simulink model "JT9D_Model_SS_test_with_alti"  (R2016b)
settings: Solver=FixedStepDiscrete  StartTime=0.0  StopTime=30.0  FixedStep=0.2  RelTol=1e-3  EnableMultiTasking=on
values from neighbouring files (symbols this model uses):
  MWS = input_set_0_0_15(MWS)    [JT9D_setup_everything_Dyn.m]    (also in JT9D_setup_everything_SS_test_with_alti.m = setup_Inputs(MWS))
undefined symbols (not defined in the file or in its folder): stripchar_TMATS
libraries: Lib_Turbo_Duct_TMATS x5, Lib_Turbo_Compressor_TMATS x3, Lib_Turbo_Shaft_TMATS x2, Lib_Turbo_TurbineNPSS_TMATS x2, Lib_Turbo_Nozzle_TMATS x2, Lib_Turbo_Ambient_TMATS x1, Lib_Turbo_Burner_TMATS x1, Lib_Turbo_Inlet_TMATS x1, Lib_Turbo_StaticCalc_TMATS x1, Lib_Turbo_SFCCalc_TMATS x1, Lib_Turbo_Splitter_TMATS x1, Lib_Solve_SSNRSolverJC_TMATS x1
settings Model: Creator=jwchapm2  LastModifiedBy=zhangshu
settings DataIOCC: LimitDataPoints=on  SaveFormat=Array
settings OptimizationCC: ExpressionDepthLimit=2147483647  LifeSpan=inf
settings DebuggingCC: UnderspecifiedInitializationDetection=Classic  MergeDetectMultiDrivingBlocksExec=none  SolverPrmCheckMsg=warning  StateNameClashWarn=warning  SFUnexpectedBacktrackingDiag=warning  SFNoUnconditionalDefaultTransitionDiag=warning  SFExecutionAtInitializationDiag=none
settings HardwareCC: ProdBitPerPointer=32  ProdBitPerSizeT=32  ProdBitPerPtrDiffT=32  ProdLargestAtomicFloat=None  ProdIntDivRoundTo=Undefined  ProdEndianess=Unspecified  ProdWordSize=32  ProdHWDeviceType=32-bit Generic
settings ModelReferenceCC: PropagateSignalLabelsOutOfModel=off
settings GRTTargetCC: TargetLangStandard=C89/C90 (ANSI)  GeneratePreprocessorConditionals=Disable all
settings ConfigComp: CovMetricSettings=dw  CovHtmlReporting=on  CovSaveCumulativeToWorkspaceVar=on  CovSaveSingleToWorkspaceVar=on  CovExternalEMLEnable=off

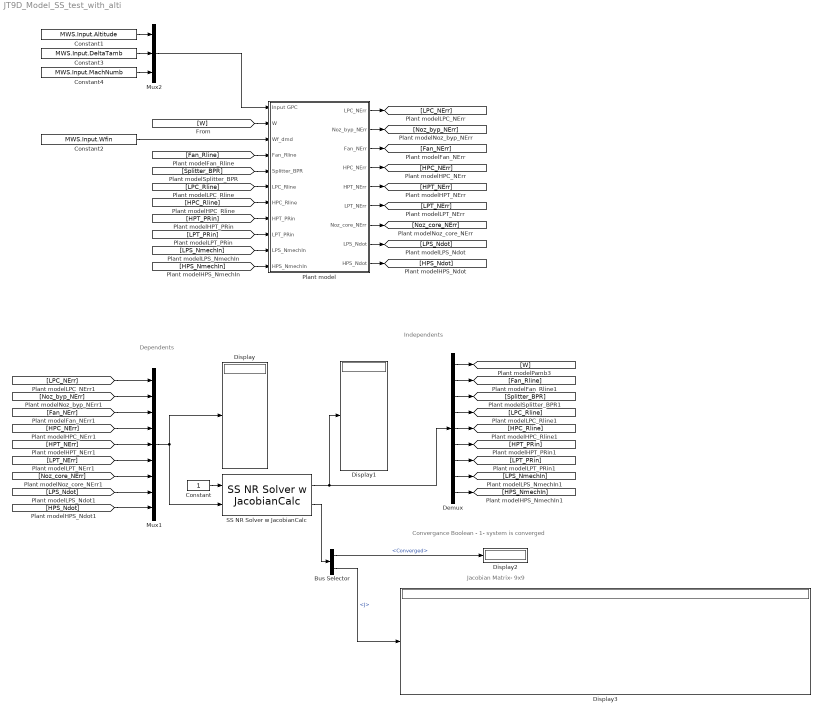
== system JT9D_Model_SS_test_with_alti ==
  note: Jacobian Matrix- 9x9
  note: Dependents
  note: Independents
  note: Convergance Boolean - 1- system is converged
  Bus Selector : BusSelector  OutputSignals=Converged,J
  Constant : Constant
  Constant1 : Constant  Value=MWS.Input.Altitude
  Constant2 : Constant  Value=MWS.Input.Wfin
  Constant3 : Constant  Value=MWS.Input.DeltaTamb
  Constant4 : Constant  Value=MWS.Input.MachNumb
  Demux : Demux  Outputs=9
  Display{,1..3} (4 alike) : Display
  Mux1 : Mux  Inputs=9
  Mux2 : Mux  Inputs=3
  Plant model : Subsystem
  SS NR Solver w JacobianCalc : Lib_Solve_SSNRSolverJC_TMATS/SS NR Solver w JacobianCalc  SJac_Per_M=0.01*[ones(size(MWS.Input.NRIC,2),1)'; -ones(size(MWS.Input.NRIC,2),1)']  SNR_IC_M=MWS.Input.NRIC  SNR_DX_M=1  SNR_Mx_M=100000  SNR_Mn_M=0.00001  SJacobianAttempts_M=20  Cond_Limits_M=0.005
  wires:
  Constant2/1 -> Plant model/3(Wf_dmd)
  [Fan_Rline] -> Plant model/4(Fan_Rline)
  [Splitter_BPR] -> Plant model/5(Splitter_BPR)
  [HPT_PRin] -> Plant model/8(HPT_PRin)
  [LPT_PRin] -> Plant model/9(LPT_PRin)
  [LPS_NmechIn] -> Plant model/10(LPS_NmechIn)
  [HPS_NmechIn] -> Plant model/11(HPS_NmechIn)
  Plant model/1(LPC_NErr) -> [LPC_NErr]
  Plant model/2(Noz_byp_NErr) -> [Noz_byp_NErr]
  Plant model/3(Fan_NErr) -> [Fan_NErr]
  Plant model/4(HPC_NErr) -> [HPC_NErr]
  Plant model/5(HPT_NErr) -> [HPT_NErr]
  Plant model/6(LPT_NErr) -> [LPT_NErr]
  Plant model/7(Noz_core_NErr) -> [Noz_core_NErr]
  Plant model/8(LPS_Ndot) -> [LPS_Ndot]
  Plant model/9(HPS_Ndot) -> [HPS_Ndot]
  Demux/1 -> [W]
  Demux/7 -> [LPT_PRin]
  Demux/5 -> [HPC_Rline]
  Demux/6 -> [HPT_PRin]
  Demux/4 -> [LPC_Rline]
  Demux/8 -> [LPS_NmechIn]
  Demux/9 -> [HPS_NmechIn]
  Demux/2 -> [Fan_Rline]
  Demux/3 -> [Splitter_BPR]
  [Fan_NErr] -> Mux1/3
  [HPC_NErr] -> Mux1/4
  [Noz_byp_NErr] -> Mux1/2
  [HPT_NErr] -> Mux1/5
  [LPC_NErr] -> Mux1/1
  [LPT_NErr] -> Mux1/6
  [Noz_core_NErr] -> Mux1/7
  SS NR Solver w JacobianCalc/2 -> Bus Selector/1
  Mux1/1 -> SS NR Solver w JacobianCalc/2, Display/1
  Bus Selector/1 -> Display2/1  "<Converged>"
  Bus Selector/2 -> Display3/1  "<J>"
  [LPS_Ndot] -> Mux1/8
  [HPS_Ndot] -> Mux1/9
  SS NR Solver w JacobianCalc/1 -> Demux/1, Display1/1
  Constant/1 -> SS NR Solver w JacobianCalc/1
  [HPC_Rline] -> Plant model/7(HPC_Rline)
  [LPC_Rline] -> Plant model/6(LPC_Rline)
  [W] -> Plant model/2(W)
  Constant1/1 -> Mux2/1
  Constant3/1 -> Mux2/2
  Constant4/1 -> Mux2/3
  Mux2/1 -> Plant model/1(Input GPC)

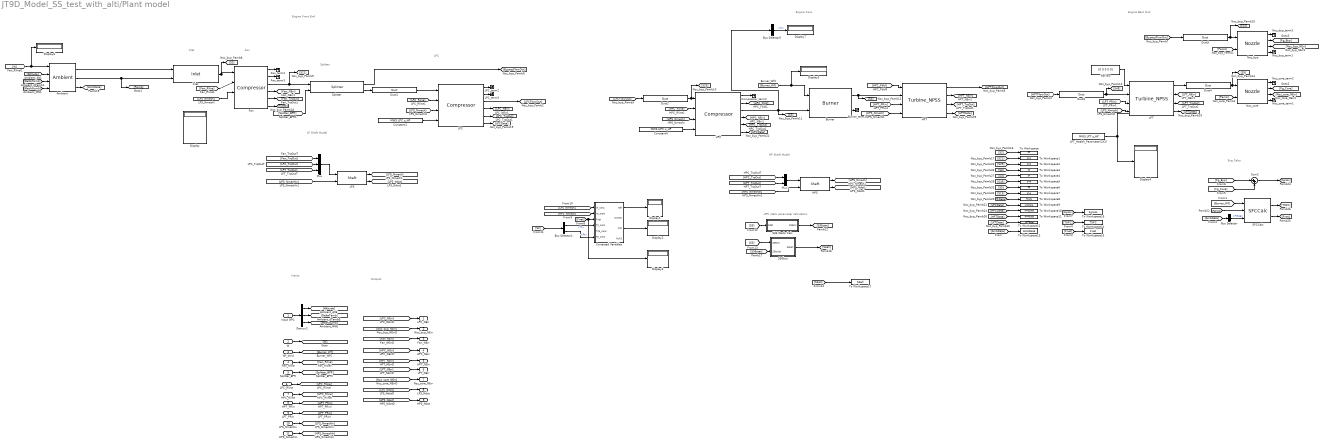
== system JT9D_Model_SS_test_with_alti/Plant model ==
  note: LP Shaft Model
  note: Inputs
  note: Outputs
  note: Engine Core
  note: HP Shaft Model
  note: Engine Back End
  note: Engine Front End
  note: Inlet
  note: Fan
  note: Splitter
  note: LPC
  note: Eng Calcs
  note: HPC static parameter calculation
  Input GPC : Inport
  W : Inport  Port=2
  Wf_dmd : Inport  Port=3
  Fan_Rline : Inport  Port=4
  Splitter_BPR : Inport  Port=5
  LPC_Rline : Inport  Port=6
  HPC_Rline : Inport  Port=7
  HPT_PRin : Inport  Port=8
  LPT_PRin : Inport  Port=9
  LPS_NmechIn : Inport  Port=10
  HPS_NmechIn : Inport  Port=11
  Ambient : Lib_Turbo_Ambient_TMATS/Ambient  X_A_AltVec_M=5000*[-1 0 1 2 3 4 5 6 7 8 9 10 12 14 16]  T_A_TsVec_M=[536.51 518.67 500.84 483.03 465.22 447.41 429.62 411.84 394.06 389.97 389.97 389.97 389.97 392.25 397.69]  T_A_PsVec_M=[17.554 14.696 12.228 10.108 8.297 6.759 5.461 4.373 3.468 2.73 2.149 1.692 1.049 0.651 0.406]  AFARc_M=0  X_A_FARVec_M=[0; 0.0050; 0.0100; 0.0150; 0.0200; 0.0250; 0.0300]  T_A_RtArray_M="[0.0686;    0.0686;    0.0686;    0.0686;    0.0686;    0.0686;    0.0686]"  Y_A_TVec_M=[300 10000]  T_A_gammaArray_M=[ 1.4 1.4 1.4 1.4 1.4 1.4 1.4; 1.4 1.4 1.4 1.4 1.4 1.4 1.4]
  Burner : Lib_Turbo_Burner_TMATS/Burner  LHVEn_M=on  LHV_M=18400  Eff_M=0.994  hFuel_M=-1200  dPnormBurner_M=MWS.Burn.dP
  Burner_term1 : Terminator
  Bus Selector : BusSelector  OutputSignals=Fdrag
  Bus Selector1 : BusSelector  OutputSignals=Tt,Pt
  Bus Selector5 : BusSelector  OutputSignals=W
  Compressor_term2 : Terminator
  Constant1 : Constant  Value=MWS.LPC.s_HP
  Constant4 : Constant  Value=MWS.HPC.s_HP
  Corrected Variables : Subsystem
  Demux2 : Demux  Outputs=3
  Display{,1..7} (8 alike) : Display
  Duct1 : Lib_Turbo_Duct_TMATS/Duct  dP_M=MWS.Duct.dP1
  Duct2 : Lib_Turbo_Duct_TMATS/Duct  dP_M=MWS.Duct.dP2
  Duct3 : Lib_Turbo_Duct_TMATS/Duct  dP_M=MWS.Duct.dP3
  Duct4 : Lib_Turbo_Duct_TMATS/Duct  dP_M=MWS.Duct.dP4
  Duct5 : Lib_Turbo_Duct_TMATS/Duct  dP_M=MWS.Duct.dP5
  Fan : Lib_Turbo_Compressor_TMATS/Compressor  X_C_RlineVec_M=MWS.FAN.RlineVec  Z_C_AlphaVec_M=1  Y_C_Map_NcVec_M=MWS.FAN.NcVec  T_C_Map_WcArray_M=MWS.FAN.WcArray  T_C_Map_PRArray_M=MWS.FAN.PRArray  T_C_Map_EffArray_M=MWS.FAN.EffArray  s_C_Nc_M=MWS.FAN.s_Nc  s_C_Wc_M=MWS.FAN.s_Wc  s_C_PR_M=MWS.FAN.s_PR  s_C_Eff_M=MWS.FAN.s_eff  SL_M=off  Scale_M=none  CBLDEN_M=off  C_CBD_M=0  C_CBFht_M=0.5  C_CBFPt_M=0.5  FBLDEN_M=off  C_FBD_M=0  C_BFht_M=0.5  C_BFPt_M=0.5  DefSMEn_M=on  SRline_M=1  X_C_Map_WcSurgeVec_M=[0 200]  T_C_Map_PRSurgeVec_M=[30 30]  iDesign_M=MWS.iDes  NcDes_M=1  EffDes_M=0.8675  PRDes_M=1.645  RlineDes_M=2.3706  FVar_M=strcat('iDes_',stripchar_TMATS(gcb),'.bin')  BlkNm_M=double(gcb)  HP_M=on
  Fan_term2 : Terminator
  Fan_term3 : Terminator
  HPC : Lib_Turbo_Compressor_TMATS/Compressor  X_C_RlineVec_M=MWS.HPC.RlineVec  Z_C_AlphaVec_M=1  Y_C_Map_NcVec_M=MWS.HPC.NcVec  T_C_Map_WcArray_M=MWS.HPC.WcArray  T_C_Map_PRArray_M=MWS.HPC.PRArray  T_C_Map_EffArray_M=MWS.HPC.EffArray  s_C_Nc_M=MWS.HPC.s_Nc  s_C_Wc_M=MWS.HPC.s_Wc  s_C_PR_M=MWS.HPC.s_PR  s_C_Eff_M=MWS.HPC.s_eff  SL_M=off  Scale_M=none  CBLDEN_M=off  C_CBD_M=0  C_CBFht_M=0.5  C_CBFPt_M=0.5  FBLDEN_M=on  C_FBD_M=MWS.HPC.Fbld  C_BFht_M=MWS.HPC.Fblde  C_BFPt_M=MWS.HPC.Fbldp  DefSMEn_M=on  SRline_M=1  X_C_Map_WcSurgeVec_M=[0 200]  T_C_Map_PRSurgeVec_M=[30 30]  iDesign_M=MWS.iDes  NcDes_M=0.995  EffDes_M=.8651  PRDes_M=5.609  RlineDes_M=2.0424  FVar_M=strcat('iDes_',stripchar_TMATS(gcb),'.bin')  BlkNm_M=double(gcb)  HP_M=on
  HPS : Lib_Turbo_Shaft_TMATS/Shaft  Shaft_Inertia_M=1000
  HPT : Lib_Turbo_TurbineNPSS_TMATS/Turbine_NPSS  X_T_Map_PRVec_M=MWS.HPT.PRVec  Y_T_Map_NcVec_M=MWS.HPT.NcVec  T_T_Map_WcArray_M=MWS.HPT.WcArray  T_T_Map_EffArray_M=MWS.HPT.EffArray  s_T_Nc_M=MWS.HPT.s_Nc  s_T_Wc_M=MWS.HPT.s_Wc  s_T_PR_M=MWS.HPT.s_PR  s_T_Eff_M=MWS.HPT.s_eff  ConfigNPSS_M=1  Scale_M=none  CFlwEn_M=on  T_CoolFlwPos_M=MWS.HPT.Cool  iDesign_M=MWS.iDes  NcDes_M=99.031  EffDes_M=.9133  PRDes_M=4.930  NDes_M=7390  FVar_M=strcat('iDes_',stripchar_TMATS(gcb),'.bin')  BlkNm_M=double(gcb)  HP_M=off
  Inlet : Lib_Turbo_Inlet_TMATS/Inlet  eRambase_M=MWS.Inlet.eRamBase  X_eRamVec_M=MWS.Inlet.eRamVec  T_eRamtbl_M=MWS.Inlet.eRamtbl
  LPC : Lib_Turbo_Compressor_TMATS/Compressor  X_C_RlineVec_M=MWS.LPC.RlineVec  Z_C_AlphaVec_M=1  Y_C_Map_NcVec_M=MWS.LPC.NcVec  T_C_Map_WcArray_M=MWS.LPC.WcArray  T_C_Map_PRArray_M=MWS.LPC.PRArray  T_C_Map_EffArray_M=MWS.LPC.EffArray  s_C_Nc_M=MWS.LPC.s_Nc  s_C_Wc_M=MWS.LPC.s_Wc  s_C_PR_M=MWS.LPC.s_PR  s_C_Eff_M=MWS.LPC.s_eff  SL_M=off  Scale_M=none  CBLDEN_M=off  C_CBD_M=0  C_CBFht_M=0.5  C_CBFPt_M=0.5  FBLDEN_M=off  C_FBD_M=0  C_BFht_M=0.5  C_BFPt_M=0.5  DefSMEn_M=on  SRline_M=1  X_C_Map_WcSurgeVec_M=[0 200]  T_C_Map_PRSurgeVec_M=[30 30]  iDesign_M=MWS.iDes  NcDes_M=0.993  EffDes_M=.8683  PRDes_M=2.488  RlineDes_M=1.7664  FVar_M=strcat('iDes_',stripchar_TMATS(gcb),'.bin')  BlkNm_M=double(gcb)  HP_M=on
  LPC_term2 : Terminator
  LPC_term3 : Terminator
  LPS : Lib_Turbo_Shaft_TMATS/Shaft  Shaft_Inertia_M=1000
  LPT : Lib_Turbo_TurbineNPSS_TMATS/Turbine_NPSS  X_T_Map_PRVec_M=MWS.LPT.PRVec  Y_T_Map_NcVec_M=MWS.LPT.NcVec  T_T_Map_WcArray_M=MWS.LPT.WcArray  T_T_Map_EffArray_M=MWS.LPT.EffArray  s_T_Nc_M=MWS.LPT.s_Nc  s_T_Wc_M=MWS.LPT.s_Wc  s_T_PR_M=MWS.LPT.s_PR  s_T_Eff_M=MWS.LPT.s_eff  ConfigNPSS_M=1  Scale_M=none  CFlwEn_M=off  T_CoolFlwPos_M=0  iDesign_M=MWS.iDes  NcDes_M=105.038  EffDes_M=.9323  PRDes_M=6.420  NDes_M=3667.6  FVar_M=strcat('iDes_',stripchar_TMATS(gcb),'.bin')  BlkNm_M=double(gcb)  HP_M=off
  LPT_Health_Parameter(2X1) : Constant  Value=MWS.LPT.s_HP
  Mux : Mux  Inputs=3
  Mux1 : Mux  Inputs=2
  NoFlow : Constant  Value=[0 0 0 0 0]
  Noz_byp : Lib_Turbo_Nozzle_TMATS/Nozzle  SWType_M=Convergent  N_TArea_M=MWS.NozB.Ath  N_EArea_M=110.7  N_FL_M=0.00  X_N_TtVec2_M=[300 2000]  T_N_TGArray_M=[1 1]  X_N_PEQPaVec_M=[0 10000]  T_N_CdThArray_M=[1 1]  T_N_CvArray_M=MWS.NozB.CvArray  CfgEn_M=off  T_N_CfgArray_M=[1 1]  X_N_FARVec_M=[0; 0.0050; 0.0100; 0.0150; 0.0200; 0.0250; 0.0300]  T_N_RtArray_M="[0.0686;    0.0686;    0.0686;    0.0686;    0.0686;    0.0686;    0.0686]"  Y_N_TtVec_M=[300 2000]  T_N_MAP_gammaArray_M=[ 1.4 1.4 1.4 1.4 1.4 1.4 1.4; 1.4 1.4 1.4 1.4 1.4 1.4 1.4]  iDesign_M=MWS.iDes  WDes_M=562.61  FVar_M=strcat('iDes_',stripchar_TMATS(gcb),'.bin')
  Noz_byp_term1 : Terminator
  Noz_byp_term3 : Terminator
  Noz_core : Lib_Turbo_Nozzle_TMATS/Nozzle  SWType_M=Convergent  N_TArea_M=MWS.Noz.Ath  N_EArea_M=110.7  N_FL_M=0.00  X_N_TtVec2_M=[300 2000]  T_N_TGArray_M=[1 1]  X_N_PEQPaVec_M=[0 10000]  T_N_CdThArray_M=[1 1]  T_N_CvArray_M=MWS.Noz.CvArray  CfgEn_M=off  T_N_CfgArray_M=[1 1]  X_N_FARVec_M=[0; 0.0050; 0.0100; 0.0150; 0.0200; 0.0250; 0.0300]  T_N_RtArray_M="[0.0686;    0.0686;    0.0686;    0.0686;    0.0686;    0.0686;    0.0686]"  Y_N_TtVec_M=[300 2000]  T_N_MAP_gammaArray_M=[ 1.4 1.4 1.4 1.4 1.4 1.4 1.4; 1.4 1.4 1.4 1.4 1.4 1.4 1.4]  iDesign_M=MWS.iDes  WDes_M=113.51  FVar_M=strcat('iDes_',stripchar_TMATS(gcb),'.bin')
  Noz_core_term1 : Terminator
  Noz_core_term2 : Terminator
  S36 Static Calc : Subsystem
  S36bus : Subsystem
  SFCCalc : Lib_Turbo_SFCCalc_TMATS/SFCCalc
  Splitter : Lib_Turbo_Splitter_TMATS/Splitter
  Sum2 : Sum  Inputs=|++
  To Workspace : ToWorkspace  VariableName=S2  SaveFormat=Timeseries  SampleTime=-1
  To Workspace1 : ToWorkspace  VariableName=S21  SaveFormat=Timeseries  SampleTime=-1
  To Workspace10 : ToWorkspace  VariableName=HPCData  SaveFormat=Timeseries  SampleTime=-1
  To Workspace11 : ToWorkspace  VariableName=HPTData  SaveFormat=Timeseries  SampleTime=-1
  To Workspace12 : ToWorkspace  VariableName=LPTData  SaveFormat=Timeseries  SampleTime=-1
  To Workspace13 : ToWorkspace  VariableName=AmbData  SaveFormat=Timeseries  SampleTime=-1
  To Workspace14 : ToWorkspace  VariableName=TSFC  SaveFormat=Timeseries  SampleTime=-1
  To Workspace15 : ToWorkspace  VariableName=Fnet  SaveFormat=Timeseries  SampleTime=-1
  To Workspace16 : ToWorkspace  VariableName=Fgross  SaveFormat=Timeseries  SampleTime=-1
  To Workspace17 : ToWorkspace  VariableName=S3all  SaveFormat=Timeseries  SampleTime=-1
  To Workspace2 : ToWorkspace  VariableName=S25  SaveFormat=Timeseries  SampleTime=-1
  To Workspace3 : ToWorkspace  VariableName=S3  SaveFormat=Timeseries  SampleTime=-1
  To Workspace4 : ToWorkspace  VariableName=S4  SaveFormat=Timeseries  SampleTime=-1
  To Workspace5 : ToWorkspace  VariableName=S45  SaveFormat=Timeseries  SampleTime=-1
  To Workspace6 : ToWorkspace  VariableName=S5  SaveFormat=Timeseries  SampleTime=-1
  To Workspace7 : ToWorkspace  VariableName=S15  SaveFormat=Timeseries  SampleTime=-1
  To Workspace8 : ToWorkspace  VariableName=FData  SaveFormat=Timeseries  SampleTime=-1
  To Workspace9 : ToWorkspace  VariableName=LPCData  SaveFormat=Timeseries  SampleTime=-1
  LPC_NErr : Outport
  Noz_byp_NErr : Outport  Port=2
  Fan_NErr : Outport  Port=3
  HPC_NErr : Outport  Port=4
  HPT_NErr : Outport  Port=5
  LPT_NErr : Outport  Port=6
  Noz_core_NErr : Outport  Port=7
  LPS_Ndot : Outport  Port=8
  HPS_Ndot : Outport  Port=9
  wires:
  Duct1/1 -> LPC/1
  Duct4/1 -> [S5], Noz_core/1
  HPC/6 -> [HPCData]
  Noz_core/4 -> Noz_core_term1/1
  [Pamb] -> Noz_core/2
  Noz_core/3 -> [Noz_core_NErr]
  Duct3/1 -> [S45], LPT/2
  Noz_core/2 -> [Fg_Core]
  Mux/1 -> LPS/1
  Mux1/1 -> HPS/1
  [LPT_TrqOut] -> Mux/3
  [Fan_TrqOut] -> Mux/1
  [HPT_TrqOut] -> Mux1/2
  [HPC_TrqOut] -> Mux1/1
  [LPC_TrqOut] -> Mux/2
  HPS/2 -> [HPS_Ndot]
  HPS/1 -> [HPS_Nmech]
  [LPS_Nmech] -> Fan/3
  [LPS_Nmech] -> LPT/4
  [HPS_NmechIn] -> HPS/2
  [HPS_Nmech] -> HPC/3
  [LPS_Nmech] -> LPC/3
  Duct2/1 -> [S25], HPC/1
  Duct5/1 -> [S15], Noz_byp/1
  LPT/2 -> [LPT_NErr]
  [LPT_PRin] -> LPT/3
  [HPS_Nmech] -> HPT/4
  LPS/2 -> [LPS_Ndot]
  LPS/1 -> [LPS_Nmech]
  [LPS_NmechIn] -> LPS/2
  Splitter/2 -> Duct1/1
  Fan/3 -> [S21], Splitter/1
  Splitter/1 -> [BypassFlowOut]
  Burner/1 -> [S4], HPT/2
  LPT/1 -> Duct4/1
  LPC/3 -> [LPCFlowOut]
  HPT/2 -> [HPT_NErr]
  [HPT_PRin] -> HPT/3
  NoFlow/1 -> LPT/1
  LPT/3 -> [LPT_TrqOut]
  HPC/1 -> Compressor_term2/1
  Noz_byp/3 -> [Noz_byp_NErr]
  [Fan_Rline] -> Fan/2
  Noz_byp/1 -> Noz_byp_term3/1
  HPT/3 -> [HPT_TrqOut]
  Noz_byp/4 -> Noz_byp_term1/1
  [Pamb] -> Noz_byp/2
  Noz_byp/2 -> [Fg_Byp]
  Burner/2 -> Burner_term1/1
  LPC/2 -> LPC_term3/1
  LPC/4 -> [LPC_NErr]
  LPC/1 -> LPC_term2/1
  LPC/5 -> [LPC_TrqOut]
  [LPC_Rline] -> LPC/2
  [Splitter_BPR] -> Splitter/2
  [HPC_Fbld] -> HPT/1
  Fan/5 -> [Fan_TrqOut]
  Fan/4 -> [Fan_NErr]
  Fan/2 -> Fan_term3/1
  Fan/6 -> [FData]
  Fan/1 -> Fan_term2/1
  HPC/5 -> [HPC_TrqOut]
  [HPC_Rline] -> HPC/2
  HPC/4 -> [HPC_NErr]
  HPC/2 -> [HPC_Fbld]
  LPC/6 -> [LPCData]
  [LPC_NErr] -> LPC_NErr/1
  [Noz_byp_NErr] -> Noz_byp_NErr/1
  [Fan_NErr] -> Fan_NErr/1
  [HPC_NErr] -> HPC_NErr/1
  [HPT_NErr] -> HPT_NErr/1
  [LPT_NErr] -> LPT_NErr/1
  [Noz_core_NErr] -> Noz_core_NErr/1
  [LPS_Ndot] -> LPS_Ndot/1
  [HPS_Ndot] -> HPS_Ndot/1
  [HPTFlowOut] -> Duct3/1
  Noz_core/1 -> Noz_core_term2/1
  [LPCFlowOut] -> Duct2/1
  HPT/1 -> [HPTFlowOut]
  [BypassFlowOut] -> Duct5/1
  HPT/4 -> [HPTData]
  LPT/4 -> [LPTData]
  [S2] -> To Workspace/1
  [S21] -> To Workspace1/1
  [S25] -> To Workspace2/1
  [S3] -> To Workspace3/1
  [S4] -> To Workspace4/1
  [S45] -> To Workspace5/1
  [S5] -> To Workspace6/1
  [S15] -> To Workspace7/1
  [FData] -> To Workspace8/1
  [LPCData] -> To Workspace9/1
  [HPCData] -> To Workspace10/1
  [HPTData] -> To Workspace11/1
  [LPTData] -> To Workspace12/1
  Inlet/1 -> Fan/1, [S2]
  LPT_Health_Parameter(2X1)/1 -> Display4/1
  [W] -> Display6/1, Ambient/1
  [Altitude] -> Ambient/2
  [DeltaTamb] -> Ambient/3
  [MachNumb] -> Ambient/4
  Ambient/3 -> [AmbData]
  Ambient/1 -> Inlet/1
  Ambient/2 -> [Pamb], Inlet/2
  Input GPC/1 -> Demux2/1
  Demux2/1 -> [Altitude]
  Demux2/2 -> [DeltaTamb]
  Demux2/3 -> [MachNumb]
  Fan_Rline/1 -> [Fan_Rline]
  HPS_NmechIn/1 -> [HPS_NmechIn]
  HPC_Rline/1 -> [HPC_Rline]
  LPT_PRin/1 -> [LPT_PRin]
  Wf_dmd/1 -> [Burner_Wf]
  Splitter_BPR/1 -> [Splitter_BPR]
  LPC_Rline/1 -> [LPC_Rline]
  HPT_PRin/1 -> [HPT_PRin]
  LPS_NmechIn/1 -> [LPS_NmechIn]
  W/1 -> [W]
  [AmbData] -> To Workspace13/1
  [Burner_Wf] -> Display5/1, Burner/1
  [AmbData] -> Bus Selector/1
  [Fg_Core] -> Sum2/2
  Sum2/1 -> [Fgross]
  Bus Selector/1 -> SFCCalc/3  "<Fdrag>"
  [Fgross] -> SFCCalc/2
  SFCCalc/2 -> [Fnet]
  SFCCalc/1 -> [TSFC]
  [Burner_Wf] -> SFCCalc/1
  [TSFC] -> To Workspace14/1
  [Fnet] -> To Workspace15/1
  [Fg_Byp] -> Sum2/1
  [Fgross] -> To Workspace16/1
  Bus Selector5/1 -> Display7/1  "<W>"
  HPC/3 -> Bus Selector5/1, [S3], Burner/2
  [Fnet] -> Display3/1, Corrected Variables/3(Fnet)
  [HPS_Nmech] -> Corrected Variables/2(nc_sens)
  [LPS_Nmech] -> Corrected Variables/1(nf_sens)
  [S2] -> Bus Selector1/1
  Bus Selector1/1 -> Corrected Variables/4(T2_sens)  "<Tt>"
  Bus Selector1/2 -> Corrected Variables/6(P2_sens)  "<Pt>"
  Corrected Variables/1(NfR) -> Display1/1
  Corrected Variables/3(FnR) -> Display2/1
  [S3] -> S36 Static Calc/1(S36t)
  S36 Static Calc/1(S36stc) -> [S36stat]
  [S3] -> S36bus/1(S36tot)
  [S36stat] -> S36bus/2(S36stat)
  S36bus/1(S36all) -> [S3all]
  [S3all] -> To Workspace17/1
  Constant4/1 -> HPC/4
  Constant1/1 -> LPC/4

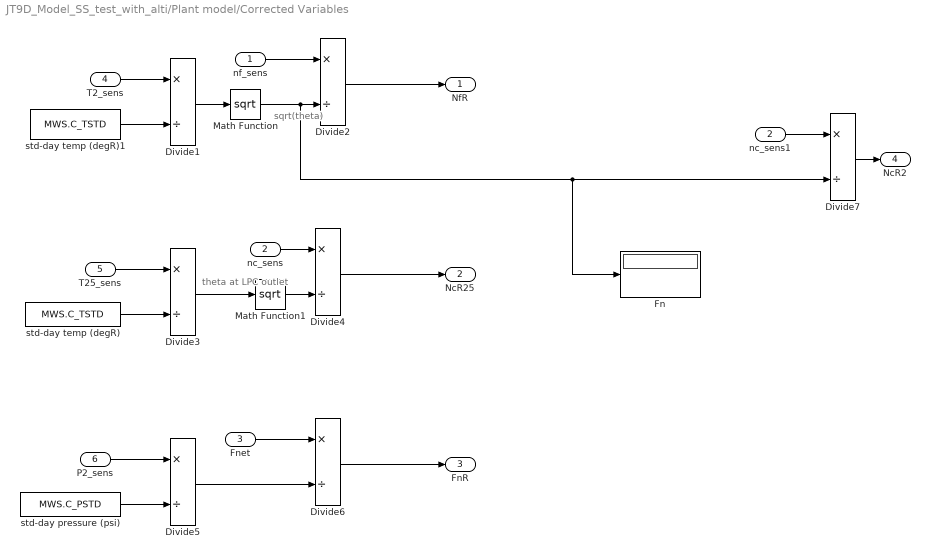
== system JT9D_Model_SS_test_with_alti/Plant model/Corrected Variables ==
  note: sqrt(theta)
  note: theta at
      | LPC outlet
  nf_sens : Inport
  nc_sens : Inport  Port=2
  Fnet : Inport  Port=3
  T2_sens : Inport  Port=4
  T25_sens : Inport  Port=5
  P2_sens : Inport  Port=6
  Divide{1..7} (7 alike) : Product  Inputs=*/
  Fn : Display
  Math Function : Math  Operator=sqrt  SaturateOnIntegerOverflow=on
  Math Function1 : Math  Operator=sqrt  SaturateOnIntegerOverflow=on
  nc_sens1 : InportShadow  Port=2
  std-day pressure (psi) : Constant  Value=MWS.C_PSTD
  std-day temp (degR) : Constant  Value=MWS.C_TSTD
  std-day temp (degR)1 : Constant  Value=MWS.C_TSTD
  NfR : Outport
  NcR25 : Outport  Port=2
  FnR : Outport  Port=3
  NcR2 : Outport  Port=4
  wires:
  Divide5/1 -> Divide6/2
  Fnet/1 -> Divide6/1
  Divide6/1 -> FnR/1
  std-day pressure (psi)/1 -> Divide5/2
  P2_sens/1 -> Divide5/1
  std-day temp (degR)/1 -> Divide3/2
  Divide1/1 -> Math Function/1
  T25_sens/1 -> Divide3/1
  std-day temp (degR)1/1 -> Divide1/2
  Divide2/1 -> NfR/1
  T2_sens/1 -> Divide1/1
  Divide3/1 -> Math Function1/1
  Math Function1/1 -> Divide4/2
  Divide4/1 -> NcR25/1
  nf_sens/1 -> Divide2/1
  Divide7/1 -> NcR2/1
  nc_sens/1 -> Divide4/1
  nc_sens1/1 -> Divide7/1
  Math Function/1 -> Fn/1, Divide7/2, Divide2/2

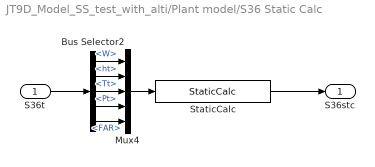
== system JT9D_Model_SS_test_with_alti/Plant model/S36 Static Calc ==
  S36t : Inport
  Bus Selector2 : BusSelector  OutputSignals=W,ht,Tt,Pt,FAR
  Mux4 : Mux  Inputs=5
  StaticCalc : Lib_Turbo_StaticCalc_TMATS/StaticCalc  ST_M=off  Ath_M=17.2  MN_M=0.3  X_FARVec_M=[0; 0.0050; 0.0100; 0.0150; 0.0200; 0.0250; 0.0300]  Y_TtVec_M=[300 10000]  T_RtArray_M="[0.0686;    0.0686;    0.0686;    0.0686;    0.0686;    0.0686;    0.0686]"  T_gammaArray_M=[ 1.4 1.4 1.4 1.4 1.4 1.4 1.4; 1.4 1.4 1.4 1.4 1.4 1.4 1.4]
  S36stc : Outport
  wires:
  Bus Selector2/4 -> Mux4/4  "<Pt>"
  Bus Selector2/2 -> Mux4/2  "<ht>"
  Bus Selector2/5 -> Mux4/5  "<FAR>"
  Bus Selector2/1 -> Mux4/1  "<W>"
  Bus Selector2/3 -> Mux4/3  "<Tt>"
  Mux4/1 -> StaticCalc/1
  StaticCalc/1 -> S36stc/1
  S36t/1 -> Bus Selector2/1

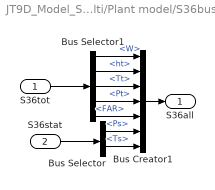
== system JT9D_Model_SS_test_with_alti/Plant model/S36bus ==
  S36tot : Inport
  S36stat : Inport  Port=2
  Bus Creator1 : BusCreator  Inputs=7
  Bus Selector : BusSelector  OutputSignals=Ps,Ts
  Bus Selector1 : BusSelector  OutputSignals=W,ht,Tt,Pt,FAR
  S36all : Outport
  wires:
  Bus Selector1/2 -> Bus Creator1/2  "<ht>"
  Bus Selector1/1 -> Bus Creator1/1  "<W>"
  Bus Selector1/5 -> Bus Creator1/5  "<FAR>"
  Bus Selector/2 -> Bus Creator1/7  "<Ts>"
  S36stat/1 -> Bus Selector/1
  S36tot/1 -> Bus Selector1/1
  Bus Selector/1 -> Bus Creator1/6  "<Ps>"
  Bus Creator1/1 -> S36all/1
  Bus Selector1/3 -> Bus Creator1/3  "<Tt>"
  Bus Selector1/4 -> Bus Creator1/4  "<Pt>"
